simulink model "generic_IsaacV5_Werkend_Clean"  (R2015a)
settings: Solver=ode45  StartTime=0.0  StopTime=inf  FixedStep=0.001  RelTol=1e-3
model workspace (MAT data in the model file):
  Gr = 10.32
  H = 0.2735
  Krf_a = 183.26
  Krr_a = 325.31
  Ksf = 12153
  Ksr = 14563
  Kwf = 0
  Kwr = 0
  L = 1.525
  Lf = 0.78
  Lr = 0.745
  M = 265
  Reff = 0.2325
  Sr = 0.6
  Tf = 1.2
  Tmax = 40
  Tr = 1.2
  g = 9.81
  mu_max = 1.5
libraries: CarMaker4SL x22, simulink x1
(part 1 of 3)
settings Model: NumberOfSteps=100  ExtModeAutoUpdateStatusClock=off  Creator=fh  LastModifiedBy=Michielvdb
settings SolverCC: ZeroCrossAlgorithm=Adaptive
settings DataIOCC: SignalLoggingSaveFormat=ModelDataLogs  SignalLoggingName=sigsOut
settings OptimizationCC: BooleanDataType=off  ExpressionDepthLimit=2147483647  InitFltsAndDblsToZero=on
settings DebuggingCC: SaveWithParameterizedLinksMsg=none  UnderspecifiedInitializationDetection=Classic  MergeDetectMultiDrivingBlocksExec=none  SignalResolutionControl=TryResolveAllWithWarning  MultiTaskDSMMsg=warning  MultiTaskCondExecSysMsg=none  FcnCallInpInsideContextMsg=UseLocalSettings  StateNameClashWarn=warning
settings HardwareCC: TargetLongLongMode=on  TargetIntDivRoundTo=Zero  TargetEndianess=LittleEndian  TargetHWDeviceType=MATLAB Host  ProdEqTarget=off
settings RTWCC: TargetLang=C++
settings CodeAppCC: MaxIdLength=63
settings GRTTargetCC: TargetFcnLib=ansi_tfl_tmw.mat  MultiInstanceERTCode=on  CodeInterfacePackaging=C++ class

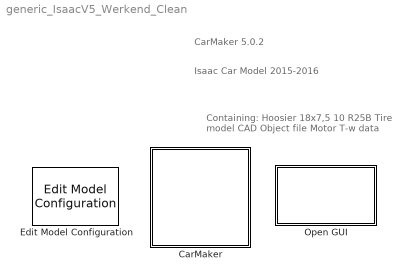
== system generic_IsaacV5_Werkend_Clean ==
  note: Isaac Car Model 2015-2016
  note: Containing:
      | Hoosier 18x7,5 10 R25B Tire model
      | CAD Object file
      | Motor T-w data
  note: CarMaker 5.0.2
  CarMaker : Subsystem  TreatAsAtomicUnit=on
      mask Display: image(imread('CarMaker4SLss.bmp'));
  Edit Model Configuration : CarMaker4SL/Edit Model Configuration
  Open GUI : Subsystem  LoadFcn=if ~length(which('cmcmd')), cmenv; end
      settings: OpenFcn=cmblockmagic('gui_fix_display'); CM_Simulink
      mask Display: image(imread('CarMakerGUI.bmp'));

== system generic_IsaacV5_Werkend_Clean/CarMaker ==
  note: PTControl: CM4SL
      | MTControl: Basic
  note: Controller
  note: Sensor output signals
  note: Sensor input signals
  CM_FIRST : Subsystem
  CM_LAST : Subsystem
  Constant2 : Constant  Value=1200  VectorParams1D=off  SampleTime=-1
  Constant3 : Constant  Value=1200  VectorParams1D=off  SampleTime=-1
  DrivMan : Subsystem
  Ground : Ground
  IPG Vehicle : Subsystem  TreatAsAtomicUnit=on
  PedalMapping : Subsystem
  Subsystem : Subsystem
  Terminator : Terminator
  TorqueVectoring : Subsystem
  Vehicle Sensors : Subsystem
  VehicleControl : Subsystem
  wires:
  DrivMan/2(DrivMan.Out) -> VehicleControl/2(DrivMan.In)
  DrivMan/1(Sync_Out) -> VehicleControl/1(Sync_In)
  CM_FIRST/2(Env.Misc) -> DrivMan/2(Env.Misc)
  CM_FIRST/1(Sync_Out) -> DrivMan/1(Sync_In)
  CM_LAST/1(Sync_Out) -> Terminator/1
  IPG Vehicle/1(Sync_Out) -> CM_LAST/1(Sync_In)
  VehicleControl/1(Sync_Out) -> IPG Vehicle/1(Sync_In)
  VehicleControl/3(VhclCtrl.Steering) -> IPG Vehicle/3(VhclCtrl.Steering)
  VehicleControl/4(Vhcl.Wheel.In) -> IPG Vehicle/4(Vhcl.Wheel.In)
  VehicleControl/5(Vhcl.Misc) -> IPG Vehicle/5(Vhcl.Misc)
  VehicleControl/6(VhclCtrl.Brake) -> IPG Vehicle/6(VhclCtrl.Brake)
  VehicleControl/7(VhclCtrl.PT) -> IPG Vehicle/7(VhclCtrl.PT)
  VehicleControl/2(Vhcl.Model.Source) -> IPG Vehicle/2(Vhcl.Model.Source)
  Ground/1 -> CM_FIRST/1(Sync_In)
  Vehicle Sensors/1(Sensor inputs1) -> Subsystem/5(SensorBus), TorqueVectoring/2(Inputs), PedalMapping/1(Sensor in)
  PedalMapping/1(T_out_Nm) -> TorqueVectoring/1(Tgevraagd)
  Constant2/1 -> Subsystem/3(WheelspeedLimitRL_RPM)
  Constant3/1 -> Subsystem/4(WheelspeedLimitRR_RPM)
  TorqueVectoring/2(Trr) -> Subsystem/2(Torque_MotRR)
  TorqueVectoring/1(Trl) -> Subsystem/1(Torque_MotRL)

== system generic_IsaacV5_Werkend_Clean/Open GUI ==
  S-Function : S-Function  FunctionName=cm_gui

== system generic_IsaacV5_Werkend_Clean/CarMaker/CM_FIRST ==
  Sync_In : Inport
  Bus Creator1 : BusCreator  Inputs=9
  Demux : Demux  Outputs=9
  Environment : S-Function  FunctionName=CM_Sfun  Parameters='Environment'
  IoIn : S-Function  FunctionName=CM_Sfun  Parameters='IoIn'
  Sync_Out : Outport
  Env.Misc : Outport  Port=2
  wires:
  Bus Creator1/1 -> Env.Misc/1
  Environment/2 -> Demux/1
  Demux/4 -> Bus Creator1/4  "Env AirHumidity"
  Demux/3 -> Bus Creator1/3  "Env AirPressure"
  Demux/2 -> Bus Creator1/2  "Env AirDensity"
  Demux/1 -> Bus Creator1/1  "Env Temperature"
  Environment/1 -> Sync_Out/1
  IoIn/1 -> Environment/1
  Sync_In/1 -> IoIn/1
  Demux/5 -> Bus Creator1/5  "Env Time"
  Demux/6 -> Bus Creator1/6  "Env SolarRadiation"
  Demux/7 -> Bus Creator1/7  "Env WindVel_tot x"
  Demux/8 -> Bus Creator1/8  "Env WindVel_tot y"
  Demux/9 -> Bus Creator1/9  "Env WindVel_tot z"

== system generic_IsaacV5_Werkend_Clean/CarMaker/CM_LAST ==
  Sync_In : Inport
  CM_User : S-Function  FunctionName=CM_Sfun  Parameters='CM_User'
  IoOut : S-Function  FunctionName=CM_Sfun  Parameters='IoOut'
  Sync_Out : Outport
  wires:
  IoOut/1 -> Sync_Out/1
  CM_User/1 -> IoOut/1
  Sync_In/1 -> CM_User/1

== system generic_IsaacV5_Werkend_Clean/CarMaker/DrivMan ==
  note: There's rarely a reason to override DrivMan signals.
      | Use the VehicleControl interface for this purpose.
  Sync_In : Inport
  Env.Misc : Inport  Port=2
  BusCreator : BusCreator  Inputs=17
  Demux : Demux  Outputs=17
  DrivMan : S-Function  FunctionName=CM_Sfun  Parameters='DrivMan'
  Sync_Out : Outport
  DrivMan.Out : Outport  Port=2
  wires:
  Demux/17 -> BusCreator/17  "DrivMan Steering Trq"
  Demux/16 -> BusCreator/16  "DrivMan Steering AngAcc"
  Demux/15 -> BusCreator/15  "DrivMan Steering AngVel"
  Demux/14 -> BusCreator/14  "DrivMan Steering Ang"
  Demux/13 -> BusCreator/13  "DrivMan Gas"
  Demux/12 -> BusCreator/12  "DrivMan Clutch"
  Demux/11 -> BusCreator/11  "DrivMan BrakePark"
  Demux/10 -> BusCreator/10  "DrivMan Brake"
  Demux/9 -> BusCreator/9  "DrivMan GearNo"
  Demux/8 -> BusCreator/8  "DrivMan SelectorCtrl"
  Demux/7 -> BusCreator/7  "DrivMan UserSignal4"
  Demux/6 -> BusCreator/6  "DrivMan UserSignal3"
  Demux/5 -> BusCreator/5  "DrivMan UserSignal2"
  Demux/4 -> BusCreator/4  "DrivMan UserSignal1"
  Demux/3 -> BusCreator/3  "DrivMan UserSignal0"
  Demux/2 -> BusCreator/2  "DrivMan Key"
  Demux/1 -> BusCreator/1  "DrivMan SST"
  Env.Misc/1 -> DrivMan/2
  Sync_In/1 -> DrivMan/1
  DrivMan/1 -> Sync_Out/1
  BusCreator/1 -> DrivMan.Out/1
  DrivMan/2 -> Demux/1

== system generic_IsaacV5_Werkend_Clean/CarMaker/IPG Vehicle ==
  Sync_In : Inport
  Vhcl.Model.Source : Inport  Port=2
  VhclCtrl.Steering : Inport  Port=3
  Vhcl.Wheel.In : Inport  Port=4
  Vhcl.Misc : Inport  Port=5
  VhclCtrl.Brake : Inport  Port=6
  VhclCtrl.PT : Inport  Port=7
  Brake : Subsystem
  CarAndTrailer : Subsystem
  PowerTrain : Subsystem
  Stop Simulation : Stop
  VehicleSource_BuiltIn : simulink/Logic and Bit Operations/Compare To Constant  relop=~=  const=1  OutDataTypeStr=boolean  ZeroCross=off
  Sync_Out : Outport
  wires:
  VhclCtrl.PT/1 -> PowerTrain/3(VhclCtrl.PT)
  Brake/1(Sync_Out) -> PowerTrain/1(Sync_In)
  CarAndTrailer/1(Sync_Out) -> Brake/1(Sync_In)
  CarAndTrailer/2(Brake.IF.In) -> Brake/2(Brake.IF.In)
  VhclCtrl.Brake/1 -> Brake/3(VhclCtrl.Brake)
  PowerTrain/1(Sync_Out) -> Sync_Out/1
  Vhcl.Misc/1 -> CarAndTrailer/4(Vhcl.Misc)
  Vhcl.Wheel.In/1 -> CarAndTrailer/3(Vhcl.Wheel.In)
  VhclCtrl.Steering/1 -> CarAndTrailer/2(VhclCtrl.Steering)
  Sync_In/1 -> CarAndTrailer/1(Sync_In)
  Vhcl.Model.Source/1 -> VehicleSource_BuiltIn/1
  VehicleSource_BuiltIn/1 -> Stop Simulation/1
  Brake/2(Vhcl.Wheel.PT) -> PowerTrain/2(Vhcl.Wheel.PT)

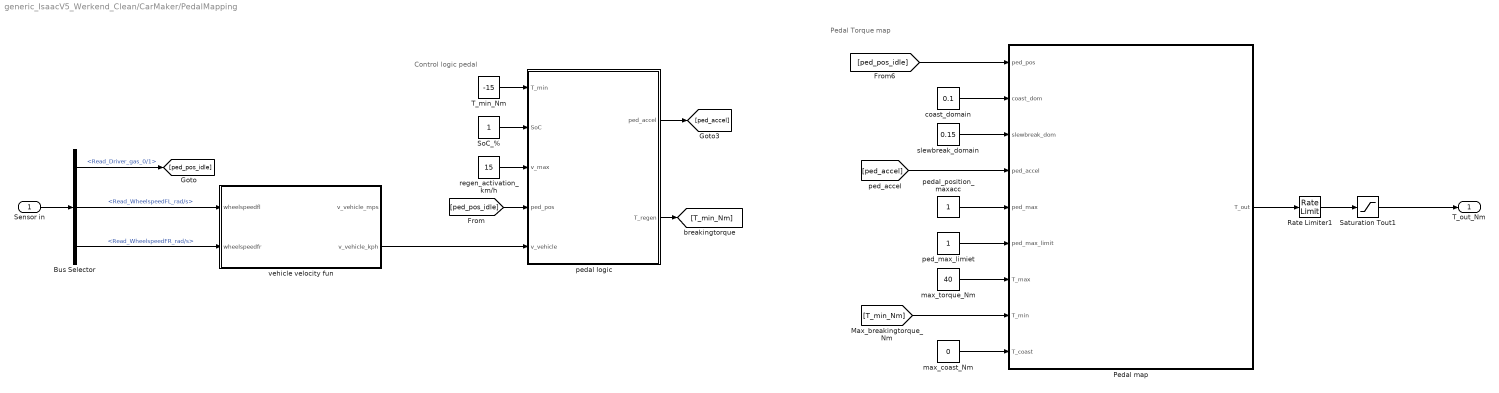
== system generic_IsaacV5_Werkend_Clean/CarMaker/PedalMapping ==
  note: Control logic pedal
  note: Pedal Torque map
  Sensor in : Inport
  Bus Selector : BusSelector  OutputSignals=Read_Driver_gas_0/1,Read_WheelspeedFL_rad/s,Read_WheelspeedFR_rad/s
  Pedal map : MATLAB Function  TreatAsAtomicUnit=on
  Rate Limiter1 : RateLimiter  RisingSlewLimit=500  FallingSlewLimit=-500
  Saturation Tout1 : Saturate  UpperLimit=40  LowerLimit=-40
  SoC_% : Constant
  T_min_Nm : Constant  Value=-15
  coast_domain : Constant  Value=0.1
  max_coast_Nm : Constant  Value=0
  max_torque_Nm : Constant  Value=40
  ped_max_limiet : Constant
  pedal logic : Stateflow chart  TreatAsAtomicUnit=on
  pedal_position_maxacc : Constant
  regen_activation_km/h : Constant  Value=15
  slewbreak_domain : Constant  Value=0.15
  vehicle velocity fun : MATLAB Function  TreatAsAtomicUnit=on
  T_out_Nm : Outport
  wires:
  [ped_accel] -> Pedal map/4(ped_accel)
  Pedal map/1(T_out) -> Rate Limiter1/1
  coast_domain/1 -> Pedal map/2(coast_dom)
  pedal_position_maxacc/1 -> Pedal map/5(ped_max)
  T_min_Nm/1 -> pedal logic/1(T_min)
  ped_max_limiet/1 -> Pedal map/6(ped_max_limit)
  [ped_pos_idle] -> Pedal map/1(ped_pos)
  slewbreak_domain/1 -> Pedal map/3(slewbreak_dom)
  [T_min_Nm] -> Pedal map/8(T_min)
  SoC_%/1 -> pedal logic/2(SoC)
  pedal logic/2(T_regen) -> [T_min_Nm]
  max_torque_Nm/1 -> Pedal map/7(T_max)
  pedal logic/1(ped_accel) -> [ped_accel]
  regen_activation_km/h/1 -> pedal logic/3(v_max)
  max_coast_Nm/1 -> Pedal map/9(T_coast)
  Sensor in/1 -> Bus Selector/1
  Bus Selector/2 -> vehicle velocity fun/1(wheelspeedfl)  "<Read_WheelspeedFL_rad/s>"
  Bus Selector/3 -> vehicle velocity fun/2(wheelspeedfr)  "<Read_WheelspeedFR_rad/s>"
  Bus Selector/1 -> [ped_pos_idle]  "<Read_Driver_gas_0/1>"
  [ped_pos_idle] -> pedal logic/4(ped_pos)
  vehicle velocity fun/2(v_vehicle_kph) -> pedal logic/5(v_vehicle)
  Rate Limiter1/1 -> Saturation Tout1/1
  Saturation Tout1/1 -> T_out_Nm/1

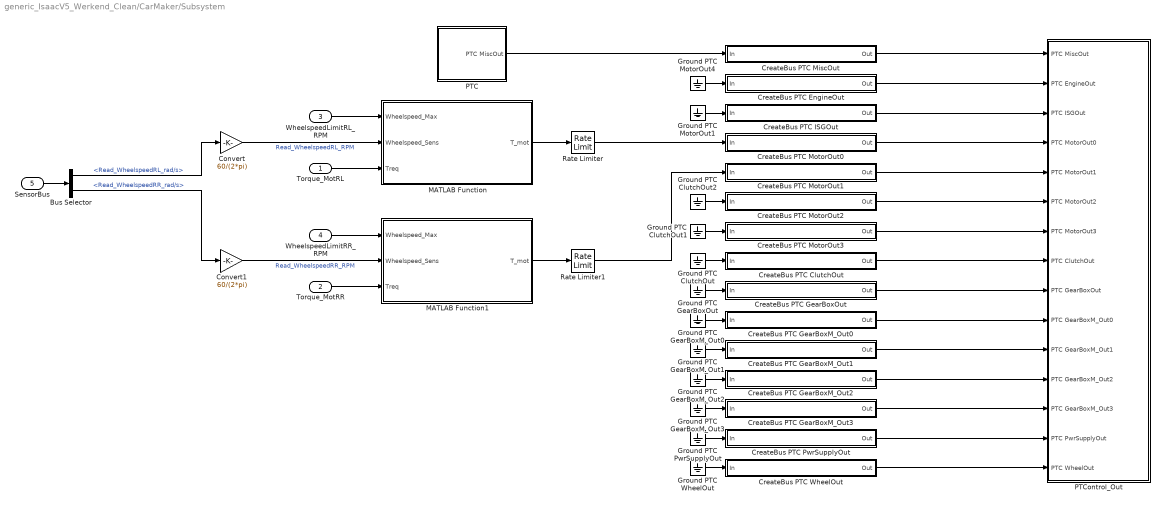
== system generic_IsaacV5_Werkend_Clean/CarMaker/Subsystem ==
  Torque_MotRL : Inport
  Torque_MotRR : Inport  Port=2
  WheelspeedLimitRL_RPM : Inport  Port=3
  WheelspeedLimitRR_RPM : Inport  Port=4
  SensorBus : Inport  Port=5
  Bus Selector : BusSelector  OutputSignals=Read_WheelspeedRL_rad/s,Read_WheelspeedRR_rad/s
  Convert : Gain  Gain=60/(2*pi)
  Convert1 : Gain  Gain=60/(2*pi)
  CreateBus PTC ClutchOut : Subsystem
  CreateBus PTC EngineOut : Subsystem
  CreateBus PTC GearBoxM_Out0 : Subsystem
  CreateBus PTC GearBoxM_Out1 : Subsystem
  CreateBus PTC GearBoxM_Out2 : Subsystem
  CreateBus PTC GearBoxM_Out3 : Subsystem
  CreateBus PTC GearBoxOut : Subsystem
  CreateBus PTC ISGOut : Subsystem
  CreateBus PTC MiscOut : Subsystem
  CreateBus PTC MotorOut0 : Subsystem
  CreateBus PTC MotorOut1 : Subsystem
  CreateBus PTC MotorOut2 : Subsystem
  CreateBus PTC MotorOut3 : Subsystem
  CreateBus PTC PwrSupplyOut : Subsystem
  CreateBus PTC WheelOut : Subsystem
  Ground PTC ClutchOut : Ground
  Ground PTC ClutchOut1 : Ground
  Ground PTC ClutchOut2 : Ground
  Ground PTC GearBoxM_Out{0..3} (4 alike) : Ground
  Ground PTC GearBoxOut : Ground
  Ground PTC MotorOut1 : Ground
  Ground PTC MotorOut4 : Ground
  Ground PTC PwrSupplyOut : Ground
  Ground PTC WheelOut : Ground
  MATLAB Function : MATLAB Function  TreatAsAtomicUnit=on
  MATLAB Function1 : MATLAB Function  TreatAsAtomicUnit=on
  PTC : Subsystem
  PTControl_Out : Subsystem
  Rate Limiter : RateLimiter  RisingSlewLimit=80  FallingSlewLimit=-80
  Rate Limiter1 : RateLimiter  RisingSlewLimit=80  FallingSlewLimit=-80
  wires:
  Ground PTC GearBoxM_Out1/1 -> CreateBus PTC GearBoxM_Out1/1(In)
  CreateBus PTC MotorOut2/1(Out) -> PTControl_Out/6(PTC MotorOut2)
  Ground PTC GearBoxOut/1 -> CreateBus PTC GearBoxOut/1(In)
  CreateBus PTC GearBoxM_Out0/1(Out) -> PTControl_Out/10(PTC GearBoxM_Out0)
  Ground PTC GearBoxM_Out0/1 -> CreateBus PTC GearBoxM_Out0/1(In)
  Ground PTC ClutchOut/1 -> CreateBus PTC ClutchOut/1(In)
  Ground PTC MotorOut4/1 -> CreateBus PTC EngineOut/1(In)
  CreateBus PTC GearBoxM_Out3/1(Out) -> PTControl_Out/13(PTC GearBoxM_Out3)
  CreateBus PTC GearBoxM_Out1/1(Out) -> PTControl_Out/11(PTC GearBoxM_Out1)
  Ground PTC GearBoxM_Out3/1 -> CreateBus PTC GearBoxM_Out3/1(In)
  Ground PTC MotorOut1/1 -> CreateBus PTC ISGOut/1(In)
  Ground PTC PwrSupplyOut/1 -> CreateBus PTC PwrSupplyOut/1(In)
  CreateBus PTC PwrSupplyOut/1(Out) -> PTControl_Out/14(PTC PwrSupplyOut)
  Ground PTC WheelOut/1 -> CreateBus PTC WheelOut/1(In)
  CreateBus PTC WheelOut/1(Out) -> PTControl_Out/15(PTC WheelOut)
  CreateBus PTC MotorOut3/1(Out) -> PTControl_Out/7(PTC MotorOut3)
  CreateBus PTC ISGOut/1(Out) -> PTControl_Out/3(PTC ISGOut)
  CreateBus PTC MotorOut1/1(Out) -> PTControl_Out/5(PTC MotorOut1)
  CreateBus PTC GearBoxM_Out2/1(Out) -> PTControl_Out/12(PTC GearBoxM_Out2)
  CreateBus PTC ClutchOut/1(Out) -> PTControl_Out/8(PTC ClutchOut)
  Ground PTC GearBoxM_Out2/1 -> CreateBus PTC GearBoxM_Out2/1(In)
  CreateBus PTC GearBoxOut/1(Out) -> PTControl_Out/9(PTC GearBoxOut)
  CreateBus PTC EngineOut/1(Out) -> PTControl_Out/2(PTC EngineOut)
  CreateBus PTC MotorOut0/1(Out) -> PTControl_Out/4(PTC MotorOut0)
  CreateBus PTC MiscOut/1(Out) -> PTControl_Out/1(PTC MiscOut)
  PTC/1(PTC MiscOut) -> CreateBus PTC MiscOut/1(In)
  Ground PTC ClutchOut1/1 -> CreateBus PTC MotorOut3/1(In)
  Ground PTC ClutchOut2/1 -> CreateBus PTC MotorOut2/1(In)
  Torque_MotRR/1 -> MATLAB Function1/3(Treq)
  Torque_MotRL/1 -> MATLAB Function/3(Treq)
  MATLAB Function/1(T_mot) -> Rate Limiter/1
  MATLAB Function1/1(T_mot) -> Rate Limiter1/1
  WheelspeedLimitRL_RPM/1 -> MATLAB Function/1(Wheelspeed_Max)
  WheelspeedLimitRR_RPM/1 -> MATLAB Function1/1(Wheelspeed_Max)
  SensorBus/1 -> Bus Selector/1
  Bus Selector/1 -> Convert/1  "<Read_WheelspeedRL_rad/s>"
  Convert/1 -> MATLAB Function/2(Wheelspeed_Sens)  "Read_WheelspeedRL_RPM"
  Bus Selector/2 -> Convert1/1  "<Read_WheelspeedRR_rad/s>"
  Convert1/1 -> MATLAB Function1/2(Wheelspeed_Sens)  "Read_WheelspeedRR_RPM"
  Rate Limiter/1 -> CreateBus PTC MotorOut0/1(In)
  Rate Limiter1/1 -> CreateBus PTC MotorOut1/1(In)

== system generic_IsaacV5_Werkend_Clean/CarMaker/TorqueVectoring ==
  Tgevraagd : Inport
  Inputs : Inport  Port=2
  2-D Lookup Table1 : Lookup_n-D  BreakpointsForDimension1=[-15,-14,-13,-12,-11,-10,-9,-8,-7,-6,-5,-4,-3,-2,-1,0,1,2,3,4,5,6,7,8,9,10,11,12,13,14,15]  BreakpointsForDimension2=[200,425,650,875,1100]  Table=reshape([-510,-510,-510,-510,-500,-500,-460,-460,-460,-420,-420,-380,-340,-270,-150,0,150,270,340,380,420,420,460,460,460,500,500,500,500,500,500,-1020,-1020,-1020,-1020,-1000,-1000,-1000,-960,-960,-920,-880,-800,-690,-540,-350,0,350,540,690,800,880,920,960,960,1000,1000,1000,1020,1020,1020,1020,-1540,-1540,-1540,-1540,-1500,-1500,-1500,-1460,-1420,-1360,-1300,-1230,-1040,-800,-500,0,500,800,1040,1230,1300,1360,1420,1460,1500,1500,1500,1540,1540,1540,1540,-2020,-2020,-2020,-2020,-1980,-1960,-1920,-1920,-1860,-1790,-1690,-1540,-1330,-960,-580,0,580,960,1330,1540,1690,1790,1860,1920,1920,1960,1980,2020,2020,2020,2020,-2500,-2500,-2500,-2440,-2420,-2420,-2380,-2300,-2250,-2180,-2000,-1800,-1540,-1150,-690,0,690,1150,1540,1800,2000,2180,2250,2300,2380,2420,2420,2440,2500,2500,2500],31,5)  InternalRulePriority=Speed  RndMeth=Simplest  InputSameDT=on
  2-D Lookup Table2 : Lookup_n-D  BreakpointsForDimension1=[-15,-14,-13,-12,-11,-10,-9,-8,-7,-6,-5,-4,-3,-2,-1,0,1,2,3,4,5,6,7,8,9,10,11,12,13,14,15]  BreakpointsForDimension2=[200,425,650,875,1100]  Table=reshape([-510,-510,-510,-510,-500,-500,-460,-460,-460,-420,-420,-380,-340,-270,-150,0,150,270,340,380,420,420,460,460,460,500,500,500,500,500,500,-1020,-1020,-1020,-1020,-1000,-1000,-1000,-960,-960,-920,-880,-800,-690,-540,-350,0,350,540,690,800,880,920,960,960,1000,1000,1000,1020,1020,1020,1020,-1540,-1540,-1540,-1540,-1500,-1500,-1500,-1460,-1420,-1360,-1300,-1230,-1040,-800,-500,0,500,800,1040,1230,1300,1360,1420,1460,1500,1500,1500,1540,1540,1540,1540,-2020,-2020,-2020,-2020,-1980,-1960,-1920,-1920,-1860,-1790,-1690,-1540,-1330,-960,-580,0,580,960,1330,1540,1690,1790,1860,1920,1920,1960,1980,2020,2020,2020,2020,-2500,-2500,-2500,-2440,-2420,-2420,-2380,-2300,-2250,-2180,-2000,-1800,-1540,-1150,-690,0,690,1150,1540,1800,2000,2180,2250,2300,2380,2420,2420,2440,2500,2500,2500],31,5)  InternalRulePriority=Speed  RndMeth=Simplest  InputSameDT=on
  Bus Selector : BusSelector  OutputSignals=Read_ay_m/s²,Read_Vhcl_Velocity,Read_Vhcl_YawRate,Read_ax_m/s²,Read_Mean_Steering_Angle_Wheels,Read_Steering_angle_rad
  Memory : Memory  X0=0.001
  Memory1 : Memory  X0=0.001
  Mu_ DroogWegdek : Constant  Value=mu_max
  PI_CONTROLLER1 : Subsystem
  Post-processor : Subsystem
  Pre-processor : Subsystem
  Signal Specification : SignalSpecification  Dimensions=1
  Signal Specification1 : SignalSpecification  Dimensions=1
  Sum4 : Sum  Inputs=|+-
  Trl : Outport
  Trr : Outport  Port=2
  wires:
  Mu_ DroogWegdek/1 -> Pre-processor/3(mu_max), Post-processor/3(mu_max)
  PI_CONTROLLER1/1(PI_out) -> Post-processor/5(Mz)  "Mz"
  Post-processor/1(Trl) -> Trl/1  "Trl"
  Post-processor/2(Trr) -> Trr/1  "Trr"
  Sum4/1 -> PI_CONTROLLER1/1(YawRate-Error)
  Memory/1 -> Pre-processor/7(alfa_r1), 2-D Lookup Table2/1
  Memory1/1 -> 2-D Lookup Table1/1, Pre-processor/8(alfa_f1)
  Pre-processor/2(alfa_f) -> Memory1/1
  Signal Specification1/1 -> Pre-processor/5(Fy_f)
  Signal Specification/1 -> Pre-processor/6(Fy_r)
  Pre-processor/3(alfa_r) -> Memory/1
  2-D Lookup Table2/1 -> Signal Specification/1
  2-D Lookup Table1/1 -> Signal Specification1/1
  Inputs/1 -> Bus Selector/1
  Tgevraagd/1 -> Post-processor/6(Tgevraagd)
  Bus Selector/6 -> ?  "<Read_Steering_angle_rad>"
  Bus Selector/4 -> Pre-processor/4(a_zwpx), Post-processor/1(ax)  "<Read_ax_m/s²>"
  Bus Selector/1 -> Post-processor/2(ay)  "<Read_ay_m/s²>"
  Bus Selector/2 -> Pre-processor/1(Vzwp), Post-processor/4(Vzwp), PI_CONTROLLER1/2(Vzwp)  "<Read_Vhcl_Velocity>"
  Post-processor/4(Wr) -> 2-D Lookup Table2/2  "Wr"
  Pre-processor/1(Yaw_ref) -> Sum4/1  "Yaw_ref"
  Bus Selector/3 -> Sum4/2  "<Read_Vhcl_YawRate>"
  Post-processor/3(Wf) -> 2-D Lookup Table1/2  "Wf"
  Bus Selector/5 -> Pre-processor/2(Stuurhoek)  "<Read_Mean_Steering_Angle_Wheels>"

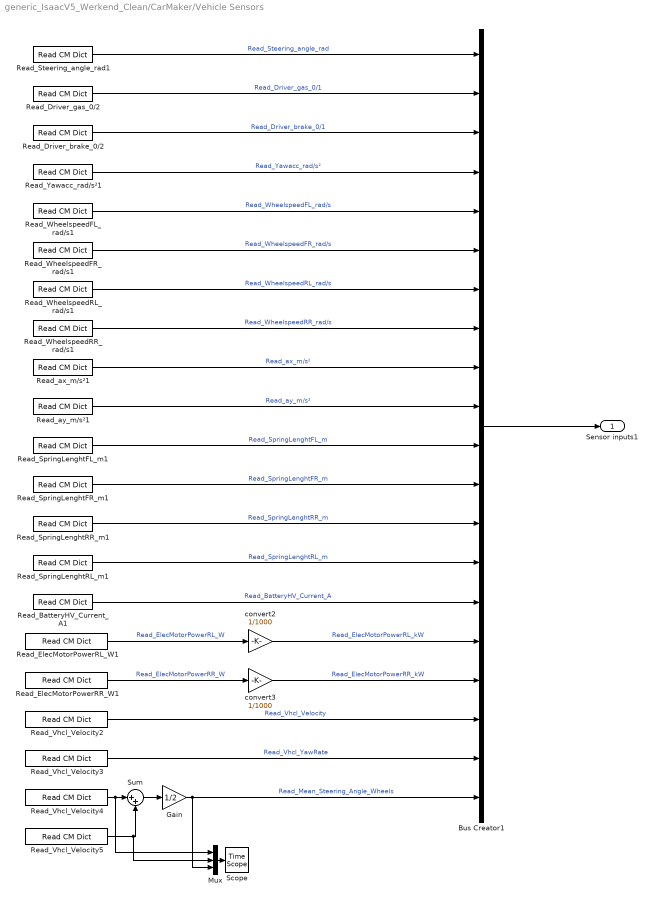
== system generic_IsaacV5_Werkend_Clean/CarMaker/Vehicle Sensors ==
  Bus Creator1 : BusCreator  Inputs=20
  Gain : Gain  Gain=1/2
  Mux : Mux  Inputs=3
  Read_BatteryHV_Current_A1 : CarMaker4SL/Read CM Dict  xname=PT.BattHV.Current  xsync=off
  Read_Driver_brake_0/2 : CarMaker4SL/Read CM Dict  xname=DM.Brake  xsync=off
  Read_Driver_gas_0/2 : CarMaker4SL/Read CM Dict  xname=DM.Gas  xsync=off
  Read_ElecMotorPowerRL_W1 : CarMaker4SL/Read CM Dict  xname=PT.Motor.PwrElec  xsync=off
  Read_ElecMotorPowerRR_W1 : CarMaker4SL/Read CM Dict  xname=PT.Motor1.PwrElec  xsync=off
  Read_SpringLenghtFL_m1 : CarMaker4SL/Read CM Dict  xname=Car.SpringFL.l  xsync=off
  Read_SpringLenghtFR_m1 : CarMaker4SL/Read CM Dict  xname=Car.SpringFR.l  xsync=off
  Read_SpringLenghtRL_m1 : CarMaker4SL/Read CM Dict  xname=Car.SpringRL.l  xsync=off
  Read_SpringLenghtRR_m1 : CarMaker4SL/Read CM Dict  xname=Car.SpringRR.l  xsync=off
  Read_Steering_angle_rad1 : CarMaker4SL/Read CM Dict  xname=Steer.WhlAng  xsync=off
  Read_Vhcl_Velocity2 : CarMaker4SL/Read CM Dict  xname=Vhcl.v  xsync=off
  Read_Vhcl_Velocity3 : CarMaker4SL/Read CM Dict  xname=Vhcl.YawRate  xsync=off
  Read_Vhcl_Velocity4 : CarMaker4SL/Read CM Dict  xname=Car.SteerAngleFL  xsync=off
  Read_Vhcl_Velocity5 : CarMaker4SL/Read CM Dict  xname=Car.SteerAngleFR  xsync=off
  Read_WheelspeedFL_rad/s1 : CarMaker4SL/Read CM Dict  xname=Vhcl.FL.rotv  xsync=off
  Read_WheelspeedFR_rad/s1 : CarMaker4SL/Read CM Dict  xname=Vhcl.FR.rotv  xsync=off
  Read_WheelspeedRL_rad/s1 : CarMaker4SL/Read CM Dict  xname=Vhcl.RL.rotv  xsync=off
  Read_WheelspeedRR_rad/s1 : CarMaker4SL/Read CM Dict  xname=Vhcl.RR.rotv  xsync=off
  Read_Yawacc_rad/s²1 : CarMaker4SL/Read CM Dict  xname=Vhcl.YawAcc  xsync=off
  Read_ax_m/s²1 : CarMaker4SL/Read CM Dict  xname=Car.ax  xsync=off
  Read_ay_m/s²1 : CarMaker4SL/Read CM Dict  xname=Car.ay  xsync=off
  Scope : TimeScope
  Sum : Sum  Inputs=|++
  convert2 : Gain  Gain=1/1000
  convert3 : Gain  Gain=1/1000
  Sensor inputs1 : Outport
  wires:
  Read_Steering_angle_rad1/1 -> Bus Creator1/1  "Read_Steering_angle_rad"
  Read_Driver_gas_0/2/1 -> Bus Creator1/2  "Read_Driver_gas_0/1"
  Read_Driver_brake_0/2/1 -> Bus Creator1/3  "Read_Driver_brake_0/1"
  Read_Yawacc_rad/s²1/1 -> Bus Creator1/4  "Read_Yawacc_rad/s²"
  Read_WheelspeedFL_rad/s1/1 -> Bus Creator1/5  "Read_WheelspeedFL_rad/s"
  Read_WheelspeedFR_rad/s1/1 -> Bus Creator1/6  "Read_WheelspeedFR_rad/s"
  Read_WheelspeedRL_rad/s1/1 -> Bus Creator1/7  "Read_WheelspeedRL_rad/s"
  Read_WheelspeedRR_rad/s1/1 -> Bus Creator1/8  "Read_WheelspeedRR_rad/s"
  Read_ax_m/s²1/1 -> Bus Creator1/9  "Read_ax_m/s²"
  Read_ay_m/s²1/1 -> Bus Creator1/10  "Read_ay_m/s²"
  Read_SpringLenghtFL_m1/1 -> Bus Creator1/11  "Read_SpringLenghtFL_m"
  Read_SpringLenghtFR_m1/1 -> Bus Creator1/12  "Read_SpringLenghtFR_m"
  Read_SpringLenghtRL_m1/1 -> Bus Creator1/14  "Read_SpringLenghtRL_m"
  Read_SpringLenghtRR_m1/1 -> Bus Creator1/13  "Read_SpringLenghtRR_m"
  Bus Creator1/1 -> Sensor inputs1/1
  Read_BatteryHV_Current_A1/1 -> Bus Creator1/15  "Read_BatteryHV_Current_A"
  Read_ElecMotorPowerRL_W1/1 -> convert2/1  "Read_ElecMotorPowerRL_W"
  Read_ElecMotorPowerRR_W1/1 -> convert3/1  "Read_ElecMotorPowerRR_W"
  convert2/1 -> Bus Creator1/16  "Read_ElecMotorPowerRL_kW"
  convert3/1 -> Bus Creator1/17  "Read_ElecMotorPowerRR_kW"
  Read_Vhcl_Velocity2/1 -> Bus Creator1/18  "Read_Vhcl_Velocity"
  Read_Vhcl_Velocity3/1 -> Bus Creator1/19  "Read_Vhcl_YawRate"
  Read_Vhcl_Velocity4/1 -> Mux/1, Sum/1
  Read_Vhcl_Velocity5/1 -> Mux/2, Sum/2
  Sum/1 -> Gain/1
  Gain/1 -> Mux/3, Bus Creator1/20  "Read_Mean_Steering_Angle_Wheels"
  Mux/1 -> Scope/1

== system generic_IsaacV5_Werkend_Clean/CarMaker/VehicleControl ==
  note: <Your model here>
  note: When implementing a vehicle control model,
      | be sure to add '-disablevehiclecontrol' to the command line arguments
      | in the CarMaker Model Configuration block.
      | Otherwise your model will possibly not see the original DrivMan signals
      | on its inputs, but those of a currently activated C-coded vehicle control model instead.
  Sync_In : Inport
  DrivMan.In : Inport  Port=2
  Bus Creator2 : BusCreator  Inputs=2
  CreateBus Vhcl.Misc : Subsystem
  CreateBus Vhcl.Wheel.In : Subsystem
  CreateBus VhclCtrl : Subsystem
  CreateBus VhclCtrl.PT : Subsystem
  CreateBus VhclCtrl.Steering : Subsystem
  Demux2 : Demux  Outputs=2
  VehicleControl : S-Function  FunctionName=CM_Sfun  Parameters='VehicleControl'
  VehicleControlUpd : S-Function  FunctionName=CM_Sfun  Parameters='VehicleControlUpd'
  Sync_Out : Outport
  Vhcl.Model.Source : Outport  Port=2
  VhclCtrl.Steering : Outport  Port=3
  Vhcl.Wheel.In : Outport  Port=4
  Vhcl.Misc : Outport  Port=5
  VhclCtrl.Brake : Outport  Port=6
  VhclCtrl.PT : Outport  Port=7
  wires:
  CreateBus VhclCtrl/1(Out) -> VehicleControlUpd/2
  VehicleControl/2 -> CreateBus VhclCtrl/1(In)
  VehicleControlUpd/2 -> Vhcl.Model.Source/1
  VehicleControlUpd/4 -> CreateBus Vhcl.Wheel.In/1(In1)
  VehicleControlUpd/5 -> CreateBus Vhcl.Misc/1(In1)
  VehicleControlUpd/6 -> Demux2/1
  VehicleControlUpd/7 -> CreateBus VhclCtrl.PT/1(In1)
  VehicleControlUpd/3 -> CreateBus VhclCtrl.Steering/1(In1)
  CreateBus Vhcl.Misc/1(Out1) -> Vhcl.Misc/1
  CreateBus Vhcl.Wheel.In/1(Out1) -> Vhcl.Wheel.In/1
  DrivMan.In/1 -> VehicleControl/2
  VehicleControl/1 -> VehicleControlUpd/1
  Sync_In/1 -> VehicleControl/1
  CreateBus VhclCtrl.PT/1(Out1) -> VhclCtrl.PT/1
  Bus Creator2/1 -> VhclCtrl.Brake/1
  CreateBus VhclCtrl.Steering/1(Out1) -> VhclCtrl.Steering/1
  VehicleControlUpd/1 -> Sync_Out/1
  Demux2/2 -> Bus Creator2/2  "VhclCtrl BrakePark"
  Demux2/1 -> Bus Creator2/1  "VhclCtrl Brake"

== system generic_IsaacV5_Werkend_Clean/CarMaker/IPG Vehicle/Brake ==
  note: <Your model here>
  note: When replacing the entire braking system,
      | be sure to add '-disablebrake' to the command line arguments
      | in the CarMaker Model Configuration block.
  Sync_In : Inport
  Brake.IF.In : Inport  Port=2
  VhclCtrl.Brake : Inport  Port=3
  Brake : S-Function  FunctionName=CM_Sfun  Parameters='Brake'
  BrakeUpd : S-Function  FunctionName=CM_Sfun  Parameters='BrakeUpd'
  BusCreator : BusCreator  Inputs=12
  CreateBus Vhcl.Wheel.PT : Subsystem
  Demux : Demux  Outputs=12
  Sync_Out : Outport
  Vhcl.Wheel.PT : Outport  Port=2
  wires:
  BrakeUpd/1 -> Sync_Out/1
  Brake/1 -> BrakeUpd/1  "Sync"
  Brake.IF.In/1 -> Brake/2
  VhclCtrl.Brake/1 -> Brake/3
  Brake/2 -> Demux/1
  BusCreator/1 -> BrakeUpd/2
  Sync_In/1 -> Brake/1
  Demux/12 -> BusCreator/12  "Brake IF Trq_Reg_trg RR"
  Demux/11 -> BusCreator/11  "Brake IF Trq_Reg_trg RL"
  Demux/10 -> BusCreator/10  "Brake IF Trq_Reg_trg FR"
  Demux/9 -> BusCreator/9  "Brake IF Trq_Reg_trg FL"
  Demux/8 -> BusCreator/8  "Brake IF Trq_PB RR"
  Demux/7 -> BusCreator/7  "Brake IF Trq_PB RL"
  Demux/6 -> BusCreator/6  "Brake IF Trq_PB FR"
  Demux/5 -> BusCreator/5  "Brake IF Trq_PB FL"
  Demux/4 -> BusCreator/4  "Brake IF Trq_WB RR"
  Demux/3 -> BusCreator/3  "Brake IF Trq_WB RL"
  Demux/2 -> BusCreator/2  "Brake IF Trq_WB FR"
  Demux/1 -> BusCreator/1  "Brake IF Trq_WB FL"
  BrakeUpd/2 -> CreateBus Vhcl.Wheel.PT/1(In)
  CreateBus Vhcl.Wheel.PT/1(Out) -> Vhcl.Wheel.PT/1

== system generic_IsaacV5_Werkend_Clean/CarMaker/IPG Vehicle/CarAndTrailer ==
  Sync_In : Inport
  VhclCtrl.Steering : Inport  Port=2
  Vhcl.Wheel.In : Inport  Port=3
  Vhcl.Misc : Inport  Port=4
  CarAndTrailerUpd : Subsystem
  Forces : Subsystem
  Ground : Ground
  Kinematics : Subsystem
  Kinetics : Subsystem
  Steering : Subsystem
  Terminator : Terminator
  Terminator1 : Terminator
  Trailer : Subsystem
  Sync_Out : Outport
  Brake.IF.In : Outport  Port=2
  wires:
  Trailer/9(Car.Hitch.FrcTrq) -> CarAndTrailerUpd/9(Car.Hitch.FrcTrq)
  Trailer/8(Vhcl.Wheel.RR) -> CarAndTrailerUpd/8(Vhcl.Wheel.RR)
  Trailer/7(Vhcl.Wheel.RL) -> CarAndTrailerUpd/7(Vhcl.Wheel.RL)
  Trailer/6(Vhcl.Wheel.FR) -> CarAndTrailerUpd/6(Vhcl.Wheel.FR)
  Trailer/5(Vhcl.Wheel.FL) -> CarAndTrailerUpd/5(Vhcl.Wheel.FL)
  Trailer/4(Vhcl.PoI) -> CarAndTrailerUpd/4(Vhcl.PoI)
  Trailer/3(Vhcl.Motion) -> CarAndTrailerUpd/3(Vhcl.Motion)
  Trailer/2(Vhcl.Steering) -> CarAndTrailerUpd/2(Vhcl.Steering)
  Trailer/1(Sync_Out) -> CarAndTrailerUpd/1(Sync_In)
  CarAndTrailerUpd/2(Brake.IF.In) -> Brake.IF.In/1
  CarAndTrailerUpd/1(Sync_Out) -> Sync_Out/1
  Vhcl.Misc/1 -> Terminator1/1
  Vhcl.Wheel.In/1 -> Terminator/1
  Kinetics/6(WheelCarrier.Misc) -> Trailer/6(WheelCarrier.Misc)
  Kinetics/5(Car.Trq_T2W) -> Trailer/5(Car.Trq_T2W)
  Steering/2(Steer.IF) -> Kinematics/2(Steer.IF)
  Kinetics/4(Car.Fr1) -> Trailer/4(Car.Fr1)
  Kinetics/3(Car.Hitch) -> Trailer/3(Car.Hitch)
  Kinetics/2(Trailer.Load) -> Trailer/2(Trailer.Load)
  VhclCtrl.Steering/1 -> Steering/2(VhclCtrl.Steering)
  Sync_In/1 -> Steering/1(Sync_In)
  Steering/1(Sync_Out) -> Kinematics/1(Sync_In)
  Kinetics/1(Sync_Out) -> Trailer/1(Sync_In)
  Ground/1 -> CarAndTrailerUpd/10(Vhcl.Fr1A)
  Forces/11(FStabi) -> Kinetics/11(FStabi)
  Forces/10(FDamp) -> Kinetics/10(FDamp)
  Forces/9(FSpring) -> Kinetics/9(FSpring)
  Forces/8(TireRR_Out) -> Kinetics/8(TireRR.Out)
  Forces/7(TireRL_Out) -> Kinetics/7(TireRL.Out)
  Forces/6(TireFR_Out) -> Kinetics/6(TireFR.Out)
  Forces/5(TireFL_Out) -> Kinetics/5(TireFL.Out)
  Forces/4(Car.Load) -> Kinetics/4(Car.Load)
  Forces/2(Car.Virtual) -> Kinetics/2(Car.Virtual)
  Kinematics/6(lSpring) -> Forces/6(lSpring)
  Kinematics/7(vDamp) -> Forces/7(vDamp)
  Forces/3(Car.Aero) -> Kinetics/3(Car.Aero)
  Forces/1(Sync_Out) -> Kinetics/1(Sync_In)
  Kinematics/5(TireRR_In) -> Forces/5(TireRR_In)
  Kinematics/4(TireRL_In) -> Forces/4(TireRL_In)
  Kinematics/3(TireFR_In) -> Forces/3(TireFR_In)
  Kinematics/2(TireFL_In) -> Forces/2(TireFL_In)
  Kinematics/1(Sync_Out) -> Forces/1(Sync_In)
  Kinematics/8(lStabi) -> Forces/8(lStabi)
  Forces/12(FBuf) -> Kinetics/12(FBuf)
  Kinematics/9(lBuf) -> Forces/9(lBuf)

== system generic_IsaacV5_Werkend_Clean/CarMaker/IPG Vehicle/PowerTrain ==
  note: When replacing the entire powertrain,
      | be sure to add '-disablepowertrain' to the command line arguments
      | in the CarMaker Model Configuration block.
  note: <Your model here>
  Sync_In : Inport
  Vhcl.Wheel.PT : Inport  Port=2
  VhclCtrl.PT : Inport  Port=3
  BusCreator : BusCreator  Inputs=40
  Demux : Demux  Outputs=40
  PowerTrain : S-Function  FunctionName=CM_Sfun  Parameters='PowerTrain'
  PowerTrainUpd : S-Function  FunctionName=CM_Sfun  Parameters='PowerTrainUpd'
  Sync_Out : Outport
  wires:
  Sync_In/1 -> PowerTrain/1
  PowerTrain/2 -> Demux/1
  PowerTrainUpd/1 -> Sync_Out/1
  PowerTrain/1 -> PowerTrainUpd/1  "Sync"
  BusCreator/1 -> PowerTrainUpd/2
  Demux/1 -> BusCreator/1  "PT IF Ignition"
  Demux/2 -> BusCreator/2  "PT IF OperationState"
  Demux/3 -> BusCreator/3  "PT IF OperationError"
  Demux/4 -> BusCreator/4  "PT IF GearNo"
  Demux/5 -> BusCreator/5  "PT IF Engine_rotv"
  Demux/6 -> BusCreator/6  "PT IF Engine_Trq (EngineControl)"
  Demux/8 -> BusCreator/8  "PT IF Trq_Supp2Bdy1 y"
  Demux/9 -> BusCreator/9  "PT IF Trq_Supp2Bdy1 z"
  Demux/10 -> BusCreator/10  "PT IF Trq_Supp2BdyEng x"
  Demux/11 -> BusCreator/11  "PT IF Trq_Supp2BdyEng y"
  Demux/12 -> BusCreator/12  "PT IF DL_iDiff_mean"
  Demux/13 -> BusCreator/13  "PT IF WFL rot"
  Demux/14 -> BusCreator/14  "PT IF WFL rotv"
  Demux/15 -> BusCreator/15  "PT IF WFL Trq_B2W"
  Demux/17 -> BusCreator/17  "PT IF WFL Trq_Supp2WC"
  Demux/18 -> BusCreator/18  "PT IF WFL Trq_BrakeReg"
  Demux/19 -> BusCreator/19  "PT IF WFL Trq_BrakeReg_max"
  Demux/20 -> BusCreator/20  "PT IF WFR rot"
  Demux/25 -> BusCreator/25  "PT IF WFR Trq_BrakeReg"
  Demux/26 -> BusCreator/26  "PT IF WFR Trq_BrakeReg_max"
  Demux/27 -> BusCreator/27  "PT IF WRL rot"
  Demux/28 -> BusCreator/28  "PT IF WRL rotv"
  Demux/31 -> BusCreator/31  "PT IF WRL Trq_Supp2WC"
  Demux/32 -> BusCreator/32  "PT IF WRL Trq_BrakeReg"
  Demux/33 -> BusCreator/33  "PT IF WRL Trq_BrakeReg_max"
  Demux/34 -> BusCreator/34  "PT IF WRR rot"
  Demux/35 -> BusCreator/35  "PT IF WRR rotv"
  Demux/36 -> BusCreator/36  "PT IF WRR Trq_B2W"
  Demux/37 -> BusCreator/37  "PT IF WRR Trq_Drive"
  Demux/39 -> BusCreator/39  "PT IF WRR Trq_BrakeReg"
  Demux/40 -> BusCreator/40  "PT IF WRR Trq_BrakeReg_max"
  VhclCtrl.PT/1 -> PowerTrain/3
  Vhcl.Wheel.PT/1 -> PowerTrain/2
  Demux/29 -> BusCreator/29  "PT IF WRL Trq_B2W"
  Demux/7 -> BusCreator/7  "PT IF Trq_Supp2Bdy1 x"
  Demux/16 -> BusCreator/16  "PT IF WFL Trq_Drive"
  Demux/21 -> BusCreator/21  "PT IF WFR rotv"
  Demux/22 -> BusCreator/22  "PT IF WFR Trq_B2W"
  Demux/23 -> BusCreator/23  "PT IF WFR Trq_Drive"
  Demux/24 -> BusCreator/24  "PT IF WFR Trq_Supp2WC"
  Demux/30 -> BusCreator/30  "PT IF WRL Trq_Drive"
  Demux/38 -> BusCreator/38  "PT IF WRR Trq_Supp2WC"

== system generic_IsaacV5_Werkend_Clean/CarMaker/Subsystem/CreateBus PTC ClutchOut ==
  In : Inport
  BusCreator : BusCreator  Inputs=3
  Demux : Demux  Outputs=3
  Out : Outport
  wires:
  In/1 -> Demux/1
  BusCreator/1 -> Out/1
  Demux/1 -> BusCreator/1  "PTC ClutchOut Pos"
  Demux/2 -> BusCreator/2  "PTC ClutchOut rotv_out_trg"
  Demux/3 -> BusCreator/3  "PTC ClutchOut Trq_out_trg"

== system generic_IsaacV5_Werkend_Clean/CarMaker/Subsystem/CreateBus PTC EngineOut ==
  In : Inport
  BusCreator : BusCreator  Inputs=5
  Demux : Demux  Outputs=5
  Out : Outport
  wires:
  In/1 -> Demux/1
  BusCreator/1 -> Out/1
  Demux/1 -> BusCreator/1  "PTC EngineOut set_ISC"
  Demux/2 -> BusCreator/2  "PTC EngineOut FuelCutOff"
  Demux/3 -> BusCreator/3  "PTC EngineOut Load"
  Demux/4 -> BusCreator/4  "PTC EngineOut Trq_trg"
  Demux/5 -> BusCreator/5  "PTC EngineOut rotv_trg"

== system generic_IsaacV5_Werkend_Clean/CarMaker/Subsystem/CreateBus PTC GearBoxM_Out0 ==
  In : Inport
  BusCreator : BusCreator  Inputs=7
  Demux : Demux  Outputs=7
  Out : Outport
  wires:
  In/1 -> Demux/1
  BusCreator/1 -> Out/1
  Demux/1 -> BusCreator/1  "PTC GearBoxM_Out0 GearNoTrg"
  Demux/2 -> BusCreator/2  "PTC GearBoxM_Out0 set_ParkBrake"
  Demux/3 -> BusCreator/3  "PTC GearBoxM_Out0 rotv_in_trg"
  Demux/4 -> BusCreator/4  "PTC GearBoxM_Out0 Trq_out_trg"
  Demux/5 -> BusCreator/5  "PTC GearBoxM_Out0 Clutch Pos"
  Demux/6 -> BusCreator/6  "PTC GearBoxM_Out0 Clutch rotv_out_trg"
  Demux/7 -> BusCreator/7  "PTC GearBoxM_Out0 Clutch Trq_out_trg"

== system generic_IsaacV5_Werkend_Clean/CarMaker/Subsystem/CreateBus PTC GearBoxM_Out1 ==
  In : Inport
  BusCreator : BusCreator  Inputs=7
  Demux : Demux  Outputs=7
  Out : Outport
  wires:
  In/1 -> Demux/1
  BusCreator/1 -> Out/1
  Demux/1 -> BusCreator/1  "PTC GearBoxM_Out1 GearNoTrg"
  Demux/2 -> BusCreator/2  "PTC GearBoxM_Out1 set_ParkBrake"
  Demux/3 -> BusCreator/3  "PTC GearBoxM_Out1 rotv_in_trg"
  Demux/4 -> BusCreator/4  "PTC GearBoxM_Out1 Trq_out_trg"
  Demux/5 -> BusCreator/5  "PTC GearBoxM_Out1 Clutch Pos"
  Demux/6 -> BusCreator/6  "PTC GearBoxM_Out1 Clutch rotv_out_trg"
  Demux/7 -> BusCreator/7  "PTC GearBoxM_Out1 Clutch Trq_out_trg"

== system generic_IsaacV5_Werkend_Clean/CarMaker/Subsystem/CreateBus PTC GearBoxM_Out2 ==
  In : Inport
  BusCreator : BusCreator  Inputs=7
  Demux : Demux  Outputs=7
  Out : Outport
  wires:
  In/1 -> Demux/1
  BusCreator/1 -> Out/1
  Demux/1 -> BusCreator/1  "PTC GearBoxM_Out2 GearNoTrg"
  Demux/2 -> BusCreator/2  "PTC GearBoxM_Out2 set_ParkBrake"
  Demux/3 -> BusCreator/3  "PTC GearBoxM_Out2 rotv_in_trg"
  Demux/4 -> BusCreator/4  "PTC GearBoxM_Out2 Trq_out_trg"
  Demux/5 -> BusCreator/5  "PTC GearBoxM_Out2 Clutch Pos"
  Demux/6 -> BusCreator/6  "PTC GearBoxM_Out2 Clutch rotv_out_trg"
  Demux/7 -> BusCreator/7  "PTC GearBoxM_Out2 Clutch Trq_out_trg"

== system generic_IsaacV5_Werkend_Clean/CarMaker/Subsystem/CreateBus PTC GearBoxM_Out3 ==
  In : Inport
  BusCreator : BusCreator  Inputs=7
  Demux : Demux  Outputs=7
  Out : Outport
  wires:
  In/1 -> Demux/1
  BusCreator/1 -> Out/1
  Demux/1 -> BusCreator/1  "PTC GearBoxM_Out3 GearNoTrg"
  Demux/2 -> BusCreator/2  "PTC GearBoxM_Out3 set_ParkBrake"
  Demux/3 -> BusCreator/3  "PTC GearBoxM_Out3 rotv_in_trg"
  Demux/4 -> BusCreator/4  "PTC GearBoxM_Out3 Trq_out_trg"
  Demux/5 -> BusCreator/5  "PTC GearBoxM_Out3 Clutch Pos"
  Demux/6 -> BusCreator/6  "PTC GearBoxM_Out3 Clutch rotv_out_trg"
  Demux/7 -> BusCreator/7  "PTC GearBoxM_Out3 Clutch Trq_out_trg"

== system generic_IsaacV5_Werkend_Clean/CarMaker/Subsystem/CreateBus PTC GearBoxOut ==
  In : Inport
  BusCreator : BusCreator  Inputs=7
  Demux : Demux  Outputs=7
  Out : Outport
  wires:
  In/1 -> Demux/1
  BusCreator/1 -> Out/1
  Demux/1 -> BusCreator/1  "PTC GearBoxOut GearNoTrg"
  Demux/2 -> BusCreator/2  "PTC GearBoxOut set_ParkBrake"
  Demux/3 -> BusCreator/3  "PTC GearBoxOut rotv_in_trg"
  Demux/4 -> BusCreator/4  "PTC GearBoxOut Trq_out_trg"
  Demux/5 -> BusCreator/5  "PTC GearBoxOut Clutch Pos"
  Demux/6 -> BusCreator/6  "PTC GearBoxOut Clutch rotv_out_trg"
  Demux/7 -> BusCreator/7  "PTC GearBoxOut Clutch Trq_out_trg"

== system generic_IsaacV5_Werkend_Clean/CarMaker/Subsystem/CreateBus PTC ISGOut ==
  In : Inport
  BusCreator : BusCreator  Inputs=3
  Demux : Demux  Outputs=3
  Out : Outport
  wires:
  In/1 -> Demux/1
  BusCreator/1 -> Out/1
  Demux/1 -> BusCreator/1  "PTC ISGOut Load"
  Demux/2 -> BusCreator/2  "PTC ISGOut Trq_trg"
  Demux/3 -> BusCreator/3  "PTC ISGOut rotv_trg"

== system generic_IsaacV5_Werkend_Clean/CarMaker/Subsystem/CreateBus PTC MiscOut ==
  In : Inport
  BusCreator : BusCreator
  Demux : Demux
  Out : Outport
  wires:
  In/1 -> Demux/1
  BusCreator/1 -> Out/1
  Demux/1 -> BusCreator/1  "PTC_Out OperationState"
  Demux/2 -> BusCreator/2  "PTC_Out OperationError"
  Demux/3 -> BusCreator/3  "PTC_Out StrategyMode"
  Demux/4 -> BusCreator/4  "PTC_Out Ignition"

== system generic_IsaacV5_Werkend_Clean/CarMaker/Subsystem/CreateBus PTC MotorOut0 ==
  In : Inport
  Bus Creator : BusCreator  Inputs=3
  BusCreator : BusCreator  Inputs=3
  Demux : Demux  Outputs=3
  "Load_mode_Not set " : Constant  Value=-99999
  "Speed_mode_notSet " : Constant  Value=-99999
  Out : Outport
  wires:
  BusCreator/1 -> Out/1
  Demux/3 -> BusCreator/3  "PTC MotorOut0 rotv_trg"
  Demux/2 -> BusCreator/2  "PTC MotorOut0 Trq_trg"
  Demux/1 -> BusCreator/1  "PTC MotorOut0 Load"
  Bus Creator/1 -> Demux/1
  "Speed_mode_notSet "/1 -> Bus Creator/3
  "Load_mode_Not set "/1 -> Bus Creator/1
  In/1 -> Bus Creator/2  "Torque_mode"

== system generic_IsaacV5_Werkend_Clean/CarMaker/Subsystem/CreateBus PTC MotorOut1 ==
  In : Inport
  Bus Creator : BusCreator  Inputs=3
  BusCreator : BusCreator  Inputs=3
  Demux : Demux  Outputs=3
  "Load_mode_Not set " : Constant  Value=-99999
  "Speed_mode_notSet " : Constant  Value=-99999
  Out : Outport
  wires:
  BusCreator/1 -> Out/1
  Demux/2 -> BusCreator/2  "PTC MotorOut1 Trq_trg"
  Demux/3 -> BusCreator/3  "PTC MotorOut1 rotv_trg"
  Demux/1 -> BusCreator/1  "PTC MotorOut1 Load"
  "Speed_mode_notSet "/1 -> Bus Creator/3
  Bus Creator/1 -> Demux/1
  "Load_mode_Not set "/1 -> Bus Creator/1
  In/1 -> Bus Creator/2

== system generic_IsaacV5_Werkend_Clean/CarMaker/Subsystem/CreateBus PTC MotorOut2 ==
  In : Inport
  BusCreator : BusCreator  Inputs=3
  Demux : Demux  Outputs=3
  Out : Outport
  wires:
  In/1 -> Demux/1
  BusCreator/1 -> Out/1
  Demux/1 -> BusCreator/1  "PTC MotorOut2 Load"
  Demux/2 -> BusCreator/2  "PTC MotorOut2 Trq_trg"
  Demux/3 -> BusCreator/3  "PTC MotorOut2 rotv_trg"

== system generic_IsaacV5_Werkend_Clean/CarMaker/Subsystem/CreateBus PTC MotorOut3 ==
  In : Inport
  BusCreator : BusCreator  Inputs=3
  Demux : Demux  Outputs=3
  Out : Outport
  wires:
  In/1 -> Demux/1
  BusCreator/1 -> Out/1
  Demux/1 -> BusCreator/1  "PTC MotorOut3 Load"
  Demux/2 -> BusCreator/2  "PTC MotorOut3 Trq_trg"
  Demux/3 -> BusCreator/3  "PTC MotorOut3 rotv_trg"

== system generic_IsaacV5_Werkend_Clean/CarMaker/Subsystem/CreateBus PTC PwrSupplyOut ==
  In : Inport
  BusCreator : BusCreator  Inputs=1
  Demux : Demux  Outputs=1
  Out : Outport
  wires:
  In/1 -> Demux/1
  BusCreator/1 -> Out/1
  Demux/1 -> BusCreator/1  "PTC PwrSupplyOut Pwr_HV1toLV_trg"

== system generic_IsaacV5_Werkend_Clean/CarMaker/Subsystem/CreateBus PTC WheelOut ==
  In : Inport
  BusCreator : BusCreator  Inputs=8
  Demux : Demux  Outputs=8
  Out : Outport
  wires:
  In/1 -> Demux/1
  BusCreator/1 -> Out/1
  Demux/1 -> BusCreator/1  "PTC WheelOut_FL Trq_BrakeReg"
  Demux/2 -> BusCreator/2  "PTC WheelOut_FL Trq_BrakeReg_max"
  Demux/3 -> BusCreator/3  "PTC WheelOut_FR Trq_BrakeReg"
  Demux/4 -> BusCreator/4  "PTC WheelOut_FR Trq_BrakeReg_max"
  Demux/5 -> BusCreator/5  "PTC WheelOut_RL Trq_BrakeReg"
  Demux/6 -> BusCreator/6  "PTC WheelOut_RL Trq_BrakeReg_max"
  Demux/7 -> BusCreator/7  "PTC WheelOut_RR Trq_BrakeReg"
  Demux/8 -> BusCreator/8  "PTC WheelOut_RR Trq_BrakeReg_max"

== system generic_IsaacV5_Werkend_Clean/CarMaker/Subsystem/PTC ==
  Constant2 : Constant
  Ground : Ground
  Mode_EngineDrive : Constant  Value=4
  Mux : Mux
  OperState_Driving : Constant  Value=4
  PTC MiscOut : Outport
  wires:
  Mux/1 -> PTC MiscOut/1
  OperState_Driving/1 -> Mux/1
  Ground/1 -> Mux/2  "OperationError"
  Mode_EngineDrive/1 -> Mux/3
  Constant2/1 -> Mux/4  "Ignition"

== system generic_IsaacV5_Werkend_Clean/CarMaker/Subsystem/PTControl_Out ==
  PTC MiscOut : Inport
  PTC EngineOut : Inport  Port=2
  PTC ISGOut : Inport  Port=3
  PTC MotorOut0 : Inport  Port=4
  PTC MotorOut1 : Inport  Port=5
  PTC MotorOut2 : Inport  Port=6
  PTC MotorOut3 : Inport  Port=7
  PTC ClutchOut : Inport  Port=8
  PTC GearBoxOut : Inport  Port=9
  PTC GearBoxM_Out0 : Inport  Port=10
  PTC GearBoxM_Out1 : Inport  Port=11
  PTC GearBoxM_Out2 : Inport  Port=12
  PTC GearBoxM_Out3 : Inport  Port=13
  PTC PwrSupplyOut : Inport  Port=14
  PTC WheelOut : Inport  Port=15
  PTControl_Out : S-Function  FunctionName=cm_ptcontrol_out
  wires:
  PTC MiscOut/1 -> PTControl_Out/1
  PTC EngineOut/1 -> PTControl_Out/2
  PTC ISGOut/1 -> PTControl_Out/3
  PTC MotorOut0/1 -> PTControl_Out/4
  PTC MotorOut1/1 -> PTControl_Out/5
  PTC MotorOut2/1 -> PTControl_Out/6
  PTC MotorOut3/1 -> PTControl_Out/7
  PTC ClutchOut/1 -> PTControl_Out/8
  PTC GearBoxOut/1 -> PTControl_Out/9
  PTC GearBoxM_Out0/1 -> PTControl_Out/10
  PTC GearBoxM_Out1/1 -> PTControl_Out/11
  PTC GearBoxM_Out2/1 -> PTControl_Out/12
  PTC GearBoxM_Out3/1 -> PTControl_Out/13
  PTC PwrSupplyOut/1 -> PTControl_Out/14
  PTC WheelOut/1 -> PTControl_Out/15

== system generic_IsaacV5_Werkend_Clean/CarMaker/TorqueVectoring/PI_CONTROLLER1 ==
  YawRate-Error : Inport
  Vzwp : Inport  Port=2
  Clamping circuit : Subsystem
  Constant : Constant  DisableCoverage=on  Value=0  OutDataTypeStr=Inherit: Inherit via back propagation  PreserveConstantTs=on
  Discrete-Time Integrator : DiscreteIntegrator  InitialConditionSetting=State (most efficient)  SampleTime=0.001  LimitOutput=on  UpperSaturationLimit=100  LowerSaturationLimit=-100
  Gain1 : Gain  Gain=1/10
  Gain2 : Gain  Gain=1/1000
  I : Product  RndMeth=Zero
  Lookup Table IifV : Lookup  InputValues=[-1 1 3 5 7 8 10 12 13 15 18 22 26 30 35 40]  Table=[50352886.7892156 50352886.7892156 5589135.45551528 1921428.35851846 975393.735493402 705695.225360316 447460.758905211 279243.629097448 236454.771525978 158654.332416002 94344.5016145154 48661.6461191947 26632.8595225856 13884.3621478696 5589.69756030357 1773.78141835761]
  Lookup Table PifV : Lookup  InputValues=[-1 1 3 5 7 8 10 12 13 15 18 22 26 30 35 40]  Table=[34635.2718980569 34635.2718980569 11590.7926431014 6627.38536761836 4783.12358808128 3932.42492202412 3196.93917901615 2407.06272090184 2253.13792386493 1777.83703218778 1346.39413645714 954.27715290151 744.973517942164 573.513734145603 406.894553185122 261.731683767634]
  P : Product  RndMeth=Zero
  Saturation : Saturate  UpperLimit=500  LowerLimit=-500
  Sum1 : Sum
  Switch : Switch  Criteria=u2 > Threshold  SaturateOnIntegerOverflow=on  InputSameDT=on
  PI_out : Outport
  wires:
  Lookup Table PifV/1 -> Gain1/1  "P_actie"
  Lookup Table IifV/1 -> Gain2/1  "I_actie"
  P/1 -> Sum1/1
  Sum1/1 -> Clamping circuit/1(preSat), Saturation/1  "Gewenste waarde"
  I/1 -> Clamping circuit/2(preIntegrator), Switch/3
  Saturation/1 -> PI_out/1  "Output controller"
  Gain1/1 -> P/1
  YawRate-Error/1 -> P/2, I/1  "Error"
  Vzwp/1 -> Lookup Table PifV/1, Lookup Table IifV/1  "V"
  Gain2/1 -> I/2
  Clamping circuit/1(Clamp) -> Switch/2
  Constant/1 -> Switch/1
  Switch/1 -> Discrete-Time Integrator/1
  Discrete-Time Integrator/1 -> Sum1/2

== system generic_IsaacV5_Werkend_Clean/CarMaker/TorqueVectoring/Post-processor ==
  ax : Inport
  ay : Inport  Port=2
  mu_max : Inport  Port=3
  Vzwp : Inport  Port=4
  Mz : Inport  Port=5
  Tgevraagd : Inport  Port=6
  Fysische beperkingen : Subsystem
  Reff : Gain  Gain=Reff
  Reff1 : Gain  Gain=Reff
  Saturation : Saturate  UpperLimit=Gr*Tmax*mu_max  LowerLimit=-Gr*Tmax*mu_max
  Saturation1 : Saturate  UpperLimit=Gr*Tmax*mu_max  LowerLimit=-Gr*Tmax*mu_max
  "Slip-controle " : MATLAB Function  TreatAsAtomicUnit=on
  Sqrt : Sqrt  SaturateOnIntegerOverflow=on
  Sqrt1 : Sqrt  SaturateOnIntegerOverflow=on
  Sum : Sum  Inputs=|++
  Sum1 : Sum  Inputs=|++
  Trl : Outport
  Trr : Outport  Port=2
  Wf : Outport  Port=3
  Wr : Outport  Port=4
  wires:
  Fysische beperkingen/2(Trr) -> Trr/1
  Fysische beperkingen/1(Trl) -> Trl/1
  Saturation1/1 -> Fysische beperkingen/2(Trr_maxB)
  Saturation/1 -> Fysische beperkingen/1(Trl_maxB)
  Tgevraagd/1 -> Fysische beperkingen/4(Tgevraagd)
  Mz/1 -> Fysische beperkingen/3(Mz)
  mu_max/1 -> "Slip-controle "/3(mu_max)
  Vzwp/1 -> "Slip-controle "/4(Vzwp)
  ax/1 -> "Slip-controle "/1(ax)
  ay/1 -> "Slip-controle "/2(ay)
  "Slip-controle "/1(A) -> Sum/1
  "Slip-controle "/3(C) -> Sum1/1
  "Slip-controle "/2(B) -> Sum/2
  "Slip-controle "/4(D) -> Sum1/2
  Sum/1 -> Sqrt/1
  Sum1/1 -> Sqrt1/1
  Sqrt1/1 -> Reff1/1
  Sqrt/1 -> Reff/1
  Reff/1 -> Saturation/1
  Reff1/1 -> Saturation1/1
  "Slip-controle "/6(Wr) -> Wr/1
  "Slip-controle "/5(Wf) -> Wf/1

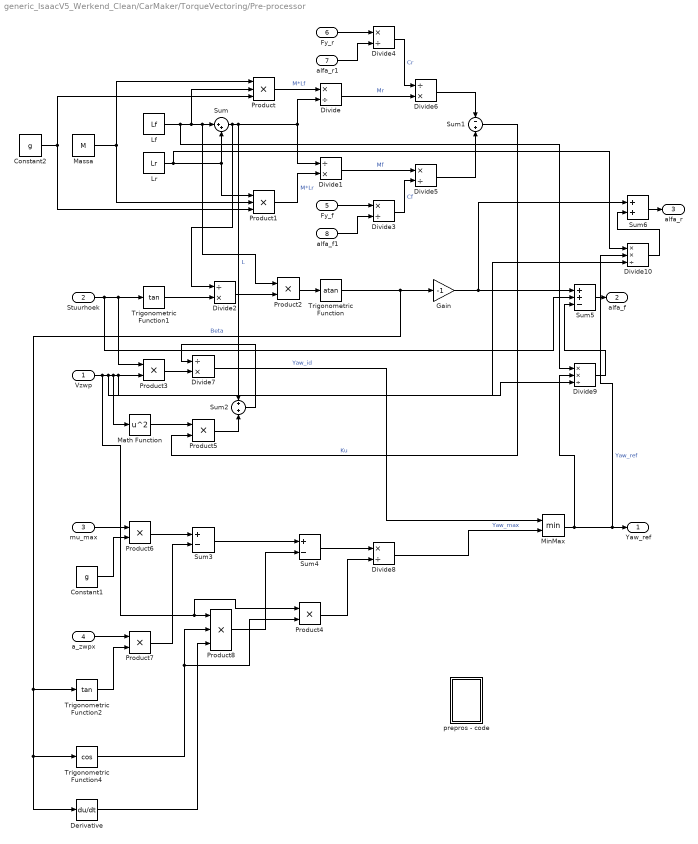
== system generic_IsaacV5_Werkend_Clean/CarMaker/TorqueVectoring/Pre-processor ==
  Vzwp : Inport
  Stuurhoek : Inport  Port=2
  mu_max : Inport  Port=3
  a_zwpx : Inport  Port=4
  Fy_f : Inport  Port=5
  Fy_r : Inport  Port=6
  alfa_r1 : Inport  Port=7
  alfa_f1 : Inport  Port=8
  Constant1 : Constant  Value=g
  Constant2 : Constant  Value=g
  Derivative : Derivative
  Divide{,3..5,8} (5 alike) : Product  Inputs=*/
  Divide{1..2,6..7} (4 alike) : Product  Inputs=/*
  Divide10 : Product  Inputs=**/
  Divide9 : Product  Inputs=**/
  Gain : Gain  Gain=-1
  Lf : Constant  Value=Lf
  Lr : Constant  Value=Lr
  Massa : Constant  Value=M
  Math Function : Math  Operator=square  SaturateOnIntegerOverflow=on
  MinMax : MinMax  Inputs=2
  Product : Product  Inputs=3
  Product1 : Product  Inputs=3
  Product{2..7} (6 alike) : Product
  Product8 : Product  Inputs=3
  Sum : Sum  Inputs=|++
  Sum1 : Sum  Inputs=-+
  Sum2 : Sum
  Sum3 : Sum  Inputs=+-
  Sum4 : Sum  Inputs=+-
  Sum5 : Sum  Inputs=++-
  Sum6 : Sum
  Trigonometric Function : Trigonometry  Operator=atan
  Trigonometric Function1 : Trigonometry  Operator=tan
  Trigonometric Function2 : Trigonometry  Operator=tan
  Trigonometric Function4 : Trigonometry  Operator=cos
  prepros - code : Subsystem
  Yaw_ref : Outport
  alfa_f : Outport  Port=2
  alfa_r : Outport  Port=3
  wires:
  Product8/1 -> Sum4/2
  Product4/1 -> Divide8/2
  Derivative/1 -> Product8/3
  MinMax/1 -> Divide9/2, Divide10/2, Yaw_ref/1  "Yaw_ref"
  Divide8/1 -> MinMax/2  "Yaw_max"
  Sum4/1 -> Divide8/1
  Fy_r/1 -> Divide4/1
  Divide4/1 -> Divide6/1  "Cr"
  Divide6/1 -> Sum1/1
  Trigonometric Function1/1 -> Divide2/2
  Divide1/1 -> Divide5/1  "Mf"
  Divide2/1 -> Product2/2
  alfa_f1/1 -> Divide3/2
  Divide/1 -> Divide6/2  "Mr"
  Trigonometric Function/1 -> Gain/1, Trigonometric Function2/1, Derivative/1, Trigonometric Function4/1  "Beta"
  alfa_r1/1 -> Divide4/2
  Product1/1 -> Divide1/2  "M*Lr"
  Lf/1 -> Divide9/1, Product/2, Product2/1, Sum/1
  Product2/1 -> Trigonometric Function/1
  Divide3/1 -> Divide5/2  "Cf"
  Massa/1 -> Product/1, Product1/2
  Product/1 -> Divide/1  "M*Lf"
  Sum/1 -> Divide/2, Divide1/1, Sum2/1, Divide2/1  "L"
  Lr/1 -> Divide10/1, Product1/1, Sum/2
  Math Function/1 -> Product5/1
  mu_max/1 -> Product6/1
  Trigonometric Function4/1 -> Product4/2, Product8/2
  Product5/1 -> Sum2/2
  Product6/1 -> Sum3/1
  Constant1/1 -> Product6/2
  Sum1/1 -> Product5/2  "Ku"
  Divide7/1 -> MinMax/1  "Yaw_id"
  Product7/1 -> Sum3/2
  Sum3/1 -> Sum4/1
  Divide5/1 -> Sum1/2
  Sum2/1 -> Divide7/1
  Vzwp/1 -> Product4/1, Product8/1, Divide9/3, Math Function/1, Divide10/3, Product3/2
  Trigonometric Function2/1 -> Product7/2
  a_zwpx/1 -> Product7/1
  Product3/1 -> Divide7/2
  Gain/1 -> Sum6/1, Sum5/1
  Divide9/1 -> Sum5/3
  Sum5/1 -> alfa_f/1
  Divide10/1 -> Sum6/2
  Sum6/1 -> alfa_r/1
  Constant2/1 -> Product1/3, Product/3
  Fy_f/1 -> Divide3/1
  Stuurhoek/1 -> Sum5/2, Product3/1, Trigonometric Function1/1

== system generic_IsaacV5_Werkend_Clean/CarMaker/VehicleControl/CreateBus Vhcl.Misc ==
  In1 : Inport
  Bus Creator5 : BusCreator  Inputs=11
  Demux5 : Demux  Outputs=11
  Out1 : Outport
  wires:
  Demux5/11 -> Bus Creator5/11  "Vhcl Wind_vel_0 z"
  Demux5/10 -> Bus Creator5/10  "Vhcl Wind_vel_0 y"
  Demux5/9 -> Bus Creator5/9  "Vhcl Wind_vel_0 x"
  Demux5/8 -> Bus Creator5/8  "Vhcl DL2BdyEng y"
  Demux5/7 -> Bus Creator5/7  "Vhcl DL2BdyEng x"
  Demux5/6 -> Bus Creator5/6  "Vhcl TrqDL2Bdy1B z"
  Demux5/5 -> Bus Creator5/5  "Vhcl TrqDL2Bdy1B y"
  Demux5/4 -> Bus Creator5/4  "Vhcl TrqDL2Bdy1B x"
  Demux5/3 -> Bus Creator5/3  "Vhcl Trq_DL2Bdy1 z"
  In1/1 -> Demux5/1
  Bus Creator5/1 -> Out1/1
  Demux5/2 -> Bus Creator5/2  "Vhcl Trq_DL2Bdy1 y"
  Demux5/1 -> Bus Creator5/1  "Vhcl Trq_DL2Bdy1 x"

== system generic_IsaacV5_Werkend_Clean/CarMaker/VehicleControl/CreateBus Vhcl.Wheel.In ==
  In1 : Inport
  Bus Creator1 : BusCreator  Inputs=12
  Demux1 : Demux  Outputs=12
  Scope{,1..5} (6 alike) : Scope
      Scope1 settings: YMin=-400  YMax=400  SaveName=ScopeData2
      Scope2 settings: YMin=-10  YMax=400  SaveName=ScopeData3
      Scope3 settings: YMin=-400  YMax=400  SaveName=ScopeData4
      Scope4 settings: YMin=-400  YMax=400  SaveName=ScopeData5
      Scope5 settings: SaveName=ScopeData6
  Out1 : Outport
  wires:
  Demux1/12 -> Scope2/1, Bus Creator1/12  "Vhcl Wheel RR rotv"
  Demux1/11 -> Scope1/1, Bus Creator1/11  "Vhcl Wheel RR Trq_DL2WC"
  Demux1/10 -> Scope/1, Bus Creator1/10  "Vhcl Wheel RR Trq_B2WC"
  Demux1/9 -> Scope3/1, Bus Creator1/9  "Vhcl Wheel RL rotv"
  Demux1/8 -> Scope4/1, Bus Creator1/8  "Vhcl Wheel RL Trq_DL2WC"
  Demux1/7 -> Scope5/1, Bus Creator1/7  "Vhcl Wheel RL Trq_B2WC"
  Demux1/6 -> Bus Creator1/6  "Vhcl Wheel FR rotv"
  Demux1/5 -> Bus Creator1/5  "Vhcl Wheel FR Trq_DL2WC"
  Demux1/4 -> Bus Creator1/4  "Vhcl Wheel FR Trq_B2WC"
  Demux1/3 -> Bus Creator1/3  "Vhcl Wheel FL rotv"
  In1/1 -> Demux1/1
  Bus Creator1/1 -> Out1/1
  Demux1/2 -> Bus Creator1/2  "Vhcl Wheel FL Trq_DL2WC"
  Demux1/1 -> Bus Creator1/1  "Vhcl Wheel FL Trq_B2WC"
